simulink model "Sampl2"  (R2021a)
settings: Solver=VariableStepAuto  StartTime=0.0  StopTime=.5  RelTol=1e-3
settings Model: Creator=arabh  LastModifiedBy=arabh

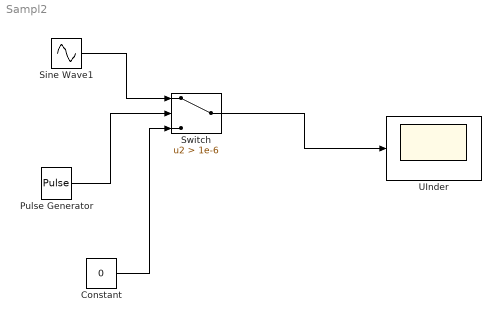
== system Sampl2 ==
  Constant : Constant  Value=0
  Pulse Generator : DiscretePulseGenerator  PulseType=Time based  Period=.01  PulseWidth=50  VectorParams1D=off
  Sine Wave1 : Sin  Frequency=20  SampleTime=0  VectorParams1D=off
  Switch : Switch  Criteria=u2 > Threshold  Threshold=1e-6
  "UInder " : Scope
  wires:
  Sine Wave1/1 -> Switch/1
  Constant/1 -> Switch/3
  Switch/1 -> "UInder "/1
  Pulse Generator/1 -> Switch/2
